simulink model "Project5_Walcher_Yilmaz_sim"  (R2022b)
settings: Solver=FixedStepDiscrete  StartTime=0.0  StopTime=Tstop  RelTol=1e-3  EnableMultiTasking=on
values from neighbouring files (symbols this model uses):
  a1 = 0.7752    [Project5_Walcher_Yilmaz.m]    (also in Sigmadelta_1bit_CIC.m)
  a2 = 0.215    [Project5_Walcher_Yilmaz.m]    (also in Sigmadelta_1bit_CIC.m)
  AMPL = 10^(A_dB/20)    (= 0.501187233627)    [Project5_Walcher_Yilmaz.m]    (also in Sigmadelta_1bit_CIC.m)
  c1 = 1    [Project5_Walcher_Yilmaz.m]    (also in Sigmadelta_1bit_CIC.m)
  dec = 64    [Project5_Walcher_Yilmaz.m]    (also in Sigmadelta_1bit_CIC.m)
  fir_num = round(fir_num*2^(nbits_coef-1))/2^(nbits_coef-1)    [Project5_Walcher_Yilmaz.m]    (also in Sigmadelta_1bit_CIC.m)
  ft_sig = tonebin/Bs    [Project5_Walcher_Yilmaz.m]    (also in Sigmadelta_1bit_CIC.m)
settings Model: Creator=ceballos  LastModifiedBy=Daniel Walcher
settings SolverCC: AlgebraicLoopSolver=TrustRegion  AutoInsertRateTranBlk=on
settings DataIOCC: LimitDataPoints=on  SaveFormat=Array  SignalLoggingSaveFormat=ModelDataLogs  ReturnWorkspaceOutputs=off
settings OptimizationCC: BooleanDataType=off  ExpressionDepthLimit=2147483647  LifeSpan=inf
settings DebuggingCC: SaveWithParameterizedLinksMsg=none  UnderspecifiedInitializationDetection=Classic  MergeDetectMultiDrivingBlocksExec=none  SignalResolutionControl=TryResolveAllWithWarning  MultiTaskDSMMsg=warning  MultiTaskCondExecSysMsg=none  FcnCallInpInsideContextMsg=warning  UnconnectedInputMsg=warning  UnconnectedOutputMsg=warning  UnconnectedLineMsg=warning  StateNameClashWarn=warning  SFUnexpectedBacktrackingDiag=warning  SFNoUnconditionalDefaultTransitionDiag=warning  SFExecutionAtInitializationDiag=none  SFMachineParentedDataDiag=warning  ArithmeticOperatorsInVariantConditions=warning
settings HardwareCC: ProdBitPerPointer=32  ProdBitPerSizeT=32  ProdBitPerPtrDiffT=32  ProdLargestAtomicFloat=None  ProdIntDivRoundTo=Undefined  ProdEndianess=Unspecified  ProdWordSize=32  ProdHWDeviceType=32-bit Generic  TargetBitPerPointer=64  TargetBitPerSizeT=64  TargetBitPerPtrDiffT=64  TargetLongLongMode=on  TargetIntDivRoundTo=Zero  TargetEndianess=LittleEndian  TargetWordSize=64  TargetHWDeviceType=MATLAB Host  ProdEqTarget=off
settings ModelReferenceCC: EnableRefExpFcnMdlSchedulingChecks=on  PropagateSignalLabelsOutOfModel=off
settings SFSimCC: SimUseLocalCustomCode=off  CustomCodeUndefinedFunction=UseInterfaceOnly
settings RTWCC: RTWUseLocalCustomCode=off
settings CodeAppCC: StateflowObjectComments=on
settings GRTTargetCC: TargetLangStandard=C89/C90 (ANSI)  CombineOutputUpdateFcns=off  GRTInterface=on
settings ConfigComp: CovMetricSettings=dw  CovSaveCumulativeToWorkspaceVar=on  CovSaveSingleToWorkspaceVar=on  CovExternalEMLEnable=off  CovSFcnEnable=off

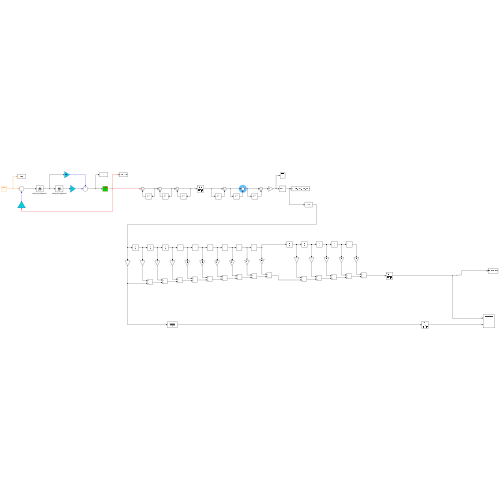
[thumbnail: Simulink's stored preview of the top-level diagram]
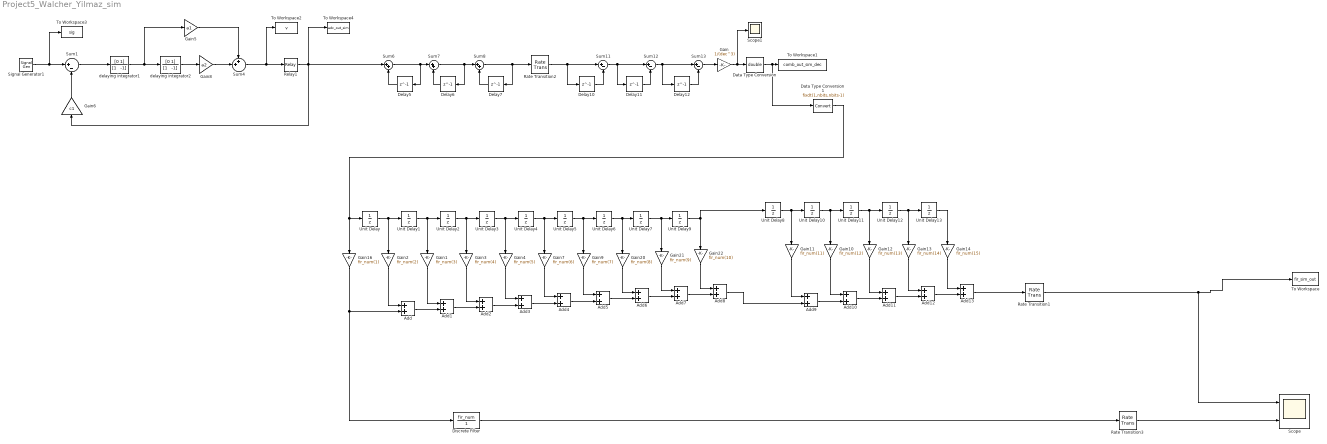
== system Project5_Walcher_Yilmaz_sim ==
  Add{,1..13} (14 alike) : Sum  OutDataTypeStr=fixdt(1,nbits_add,nbits+xbits-1)
  Data Type Conversion : DataTypeConversion  OutDataTypeStr=double  SaturateOnIntegerOverflow=off  RndMeth=Floor
  Data Type Conversion1 : DataTypeConversion  OutDataTypeStr=fixdt(1,nbits,nbits-1)  SaturateOnIntegerOverflow=off  RndMeth=Floor
  Delay{5..7,10..12} (6 alike) : Delay  DelayLength=1  InitialCondition=0
  Discrete Filter : DiscreteFilter  Numerator=fir_num  Denominator=1
  Gain : Gain  Gain=1/(dec^3)
  Gain1 : Gain  Gain=fir_num(3)  ParamDataTypeStr=fixdt(1,nbits_coef,nbits_coef-1)  OutDataTypeStr=fixdt(1,nbits+xbits,nbits+xbits-1)
  Gain10 : Gain  Gain=fir_num(12)  ParamDataTypeStr=fixdt(1,nbits_coef,nbits_coef-1)  OutDataTypeStr=fixdt(1,nbits+xbits,nbits+xbits-1)
  Gain11 : Gain  Gain=fir_num(11)  ParamDataTypeStr=fixdt(1,nbits_coef,nbits_coef-1)  OutDataTypeStr=fixdt(1,nbits+xbits,nbits+xbits-1)
  Gain12 : Gain  Gain=fir_num(13)  ParamDataTypeStr=fixdt(1,nbits_coef,nbits_coef-1)  OutDataTypeStr=fixdt(1,nbits+xbits,nbits+xbits-1)
  Gain13 : Gain  Gain=fir_num(14)  ParamDataTypeStr=fixdt(1,nbits_coef,nbits_coef-1)  OutDataTypeStr=fixdt(1,nbits+xbits,nbits+xbits-1)
  Gain14 : Gain  Gain=fir_num(15)  ParamDataTypeStr=fixdt(1,nbits_coef,nbits_coef-1)  OutDataTypeStr=fixdt(1,nbits+xbits,nbits+xbits-1)
  Gain16 : Gain  Gain=fir_num(1)  ParamDataTypeStr=fixdt(1,nbits_coef,nbits_coef-1)  OutDataTypeStr=fixdt(1,nbits+xbits,nbits+xbits-1)
  Gain2 : Gain  Gain=fir_num(2)  ParamDataTypeStr=fixdt(1,nbits_coef,nbits_coef-1)  OutDataTypeStr=fixdt(1,nbits+xbits,nbits+xbits-1)
  Gain20 : Gain  Gain=fir_num(8)  ParamDataTypeStr=fixdt(1,nbits_coef,nbits_coef-1)  OutDataTypeStr=fixdt(1,nbits+xbits,nbits+xbits-1)
  Gain21 : Gain  Gain=fir_num(9)  ParamDataTypeStr=fixdt(1,nbits_coef,nbits_coef-1)  OutDataTypeStr=fixdt(1,nbits+xbits,nbits+xbits-1)
  Gain22 : Gain  Gain=fir_num(10)  ParamDataTypeStr=fixdt(1,nbits_coef,nbits_coef-1)  OutDataTypeStr=fixdt(1,nbits+xbits,nbits+xbits-1)
  Gain3 : Gain  Gain=fir_num(4)  ParamDataTypeStr=fixdt(1,nbits_coef,nbits_coef-1)  OutDataTypeStr=fixdt(1,nbits+xbits,nbits+xbits-1)
  Gain4 : Gain  Gain=fir_num(5)  ParamDataTypeStr=fixdt(1,nbits_coef,nbits_coef-1)  OutDataTypeStr=fixdt(1,nbits+xbits,nbits+xbits-1)
  Gain5 : Gain  Gain=a1  SaturateOnIntegerOverflow=on  OutDataTypeStr=Inherit: Same as input  ParamDataTypeStr=Inherit: Same as input
  Gain6 : Gain  Gain=c1  SaturateOnIntegerOverflow=on  OutDataTypeStr=Inherit: Same as input  ParamDataTypeStr=Inherit: Same as input
  Gain7 : Gain  Gain=fir_num(6)  ParamDataTypeStr=fixdt(1,nbits_coef,nbits_coef-1)  OutDataTypeStr=fixdt(1,nbits+xbits,nbits+xbits-1)
  Gain8 : Gain  Gain=a2  SaturateOnIntegerOverflow=on  OutDataTypeStr=Inherit: Same as input  ParamDataTypeStr=Inherit: Same as input
  Gain9 : Gain  Gain=fir_num(7)  ParamDataTypeStr=fixdt(1,nbits_coef,nbits_coef-1)  OutDataTypeStr=fixdt(1,nbits+xbits,nbits+xbits-1)
  Rate Transition1 : RateTransition  OutPortSampleTimeOpt=Multiple of input port sample time  OutPortSampleTimeMultiple=4
  Rate Transition2 : RateTransition  OutPortSampleTimeOpt=Multiple of input port sample time  OutPortSampleTimeMultiple=dec
  Rate Transition3 : RateTransition  OutPortSampleTimeOpt=Multiple of input port sample time  OutPortSampleTimeMultiple=4
  Relay1 : Relay  OffSwitchValue=-eps  OffOutputValue=-1
  Scope : Scope  NumInputPorts=2
  Scope1 : Scope
  Signal Generator1 : SignalGenerator  Amplitude=AMPL  Frequency=ft_sig
  Sum1 : Sum  Inputs=|+-  InputSameDT=on  SaturateOnIntegerOverflow=on  OutDataTypeStr=Inherit: Same as first input
  Sum11 : Sum  Inputs=|+-  AccumDataTypeStr=fixdt(1,19,0)  OutDataTypeStr=Inherit: Same as accumulator
  Sum12 : Sum  Inputs=|+-  AccumDataTypeStr=fixdt(1,19,0)  OutDataTypeStr=Inherit: Same as accumulator
  Sum13 : Sum  Inputs=|+-  AccumDataTypeStr=fixdt(1,19,0)  OutDataTypeStr=Inherit: Same as accumulator
  Sum4 : Sum  Inputs=++|  InputSameDT=on  SaturateOnIntegerOverflow=on  OutDataTypeStr=Inherit: Same as first input
  Sum6 : Sum  Inputs=|++  AccumDataTypeStr=fixdt(1,19,0)  OutDataTypeStr=Inherit: Same as accumulator
  Sum7 : Sum  Inputs=|++  AccumDataTypeStr=fixdt(1,19,0)  OutDataTypeStr=Inherit: Same as accumulator
  Sum8 : Sum  Inputs=|++  AccumDataTypeStr=fixdt(1,19,0)  OutDataTypeStr=Inherit: Same as accumulator
  To Workspace : ToWorkspace  VariableName=fir_sim_out  SampleTime=-1
  To Workspace1 : ToWorkspace  VariableName=comb_out_sim_dec  SampleTime=-1
  To Workspace2 : ToWorkspace  VariableName=v  SampleTime=1
  To Workspace3 : ToWorkspace  VariableName=sig  SampleTime=1
  To Workspace4 : ToWorkspace  VariableName=adc_out_sim  SampleTime=1
  Unit Delay{,1..13} (14 alike) : UnitDelay  SampleTime=-1  HasFrameUpgradeWarning=on
  "delaying integrator1 " : DiscreteFilter  Numerator=[0 1]  Denominator="[1   -1]"  SampleTime=1
  "delaying integrator2 " : DiscreteFilter  Numerator=[0 1]  Denominator="[1   -1]"  SampleTime=1
  wires:
  "delaying integrator1 "/1 -> "delaying integrator2 "/1, Gain5/1
  Sum4/1 -> Relay1/1, To Workspace2/1
  Sum1/1 -> "delaying integrator1 "/1
  "delaying integrator2 "/1 -> Gain8/1
  Gain5/1 -> Sum4/1
  Gain8/1 -> Sum4/2
  Signal Generator1/1 -> Sum1/1, To Workspace3/1
  Gain6/1 -> Sum1/2
  Sum12/1 -> Sum13/1, Delay12/1
  Sum11/1 -> Delay11/1, Sum12/1
  Delay11/1 -> Sum12/2
  Sum7/1 -> Sum8/1, Delay6/1
  Sum6/1 -> Sum7/1, Delay5/1
  Delay10/1 -> Sum11/2
  Sum8/1 -> Rate Transition2/1, Delay7/1
  Rate Transition2/1 -> Delay10/1, Sum11/1
  Delay6/1 -> Sum7/2
  Delay12/1 -> Sum13/2
  Delay7/1 -> Sum8/2
  Delay5/1 -> Sum6/2
  Sum13/1 -> Gain/1
  Gain/1 -> Scope1/1, Data Type Conversion/1
  Rate Transition1/1 -> Scope/1, To Workspace/1
  Gain11/1 -> Add9/1
  Unit Delay10/1 -> Gain10/1, Unit Delay11/1
  Unit Delay13/1 -> Gain14/1
  Add10/1 -> Add11/2
  Unit Delay8/1 -> Gain11/1, Unit Delay10/1
  Unit Delay12/1 -> Gain13/1, Unit Delay13/1
  Gain10/1 -> Add10/1
  Add9/1 -> Add10/2
  Unit Delay11/1 -> Gain12/1, Unit Delay12/1
  Gain14/1 -> Add13/1
  Add12/1 -> Add13/2
  Add8/1 -> Add9/2
  Gain9/1 -> Add5/1
  Gain3/1 -> Add2/1
  Add/1 -> Add1/2
  Unit Delay9/1 -> Gain22/1, Unit Delay8/1
  Gain1/1 -> Add1/1
  Gain22/1 -> Add8/1
  Add7/1 -> Add8/2
  Gain7/1 -> Add4/1
  Unit Delay2/1 -> Gain3/1, Unit Delay3/1
  Add1/1 -> Add2/2
  Gain12/1 -> Add11/1
  Gain4/1 -> Add3/1
  Unit Delay7/1 -> Gain21/1, Unit Delay9/1
  Unit Delay1/1 -> Gain1/1, Unit Delay2/1
  Gain21/1 -> Add7/1
  Gain16/1 -> Discrete Filter/1, Add/2
  Add4/1 -> Add5/2
  Unit Delay4/1 -> Gain7/1, Unit Delay5/1
  Gain2/1 -> Add/1
  Gain20/1 -> Add6/1
  Add3/1 -> Add4/2
  Add5/1 -> Add6/2
  Add2/1 -> Add3/2
  Gain13/1 -> Add12/1
  Add11/1 -> Add12/2
  Add6/1 -> Add7/2
  Unit Delay/1 -> Gain2/1, Unit Delay1/1
  Unit Delay3/1 -> Gain4/1, Unit Delay4/1
  Unit Delay6/1 -> Gain20/1, Unit Delay7/1
  Unit Delay5/1 -> Gain9/1, Unit Delay6/1
  Discrete Filter/1 -> Rate Transition3/1
  Rate Transition3/1 -> Scope/2
  Relay1/1 -> Sum6/1, To Workspace4/1, Gain6/1
  Data Type Conversion/1 -> Data Type Conversion1/1, To Workspace1/1
  Data Type Conversion1/1 -> Unit Delay/1, Gain16/1
  Add13/1 -> Rate Transition1/1
